simulink model "PEM_cell_validate_dynamic"  (R2025b)
settings: Solver=ode23t  StartTime=0.0  StopTime=29988  RelTol=1e-3
values from neighbouring files (symbols this model uses):
  Active_Area = 17.64    [PV_PEM_direct_battery_active.m]    (also in PV_PEM_direct_battery_passive.m; PV_PEM_indirect_battery.m; PV_PEM_reconfigurable_battery.m; Sim_vs_meas_dynamic.m)
  Input_Time = T{:,5}    [Sim_vs_meas_dynamic.m]
  Input_Voltage = T{:,16}    [Sim_vs_meas_dynamic.m]
  Ra = 0.00177    [PV_PEM_direct_battery_active.m]    (also in PV_PEM_direct_battery_passive.m; PV_PEM_indirect_battery.m; PV_PEM_reconfigurable_battery.m; Sim_vs_meas_dynamic.m)
  Rc = 0.0005    [PV_PEM_direct_battery_active.m]    (also in PV_PEM_direct_battery_passive.m; PV_PEM_indirect_battery.m; PV_PEM_reconfigurable_battery.m; Sim_vs_meas_dynamic.m)
  Rint = 0.008673    [PV_PEM_direct_battery_active.m]    (also in PV_PEM_direct_battery_passive.m; PV_PEM_indirect_battery.m; PV_PEM_reconfigurable_battery.m; Sim_vs_meas_dynamic.m)
  Vint = 1.475841    [PV_PEM_direct_battery_active.m]    (also in PV_PEM_direct_battery_passive.m; PV_PEM_indirect_battery.m; PV_PEM_reconfigurable_battery.m; Sim_vs_meas_dynamic.m)
libraries: fl_lib x15, nesl_utility x9, simulink x2
settings Model: Creator=hanna  LastModifiedBy=hanna
settings DataIOCC: SignalLogging=off  StreamToWks=off  ReturnWorkspaceOutputs=off
settings DebuggingCC: SaveWithParameterizedLinksMsg=none

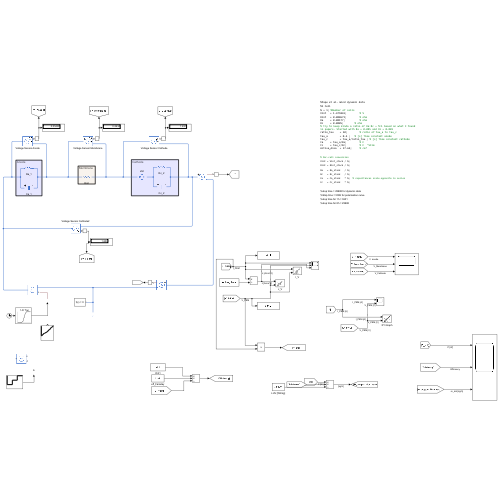
[thumbnail: Simulink's stored preview of the top-level diagram]
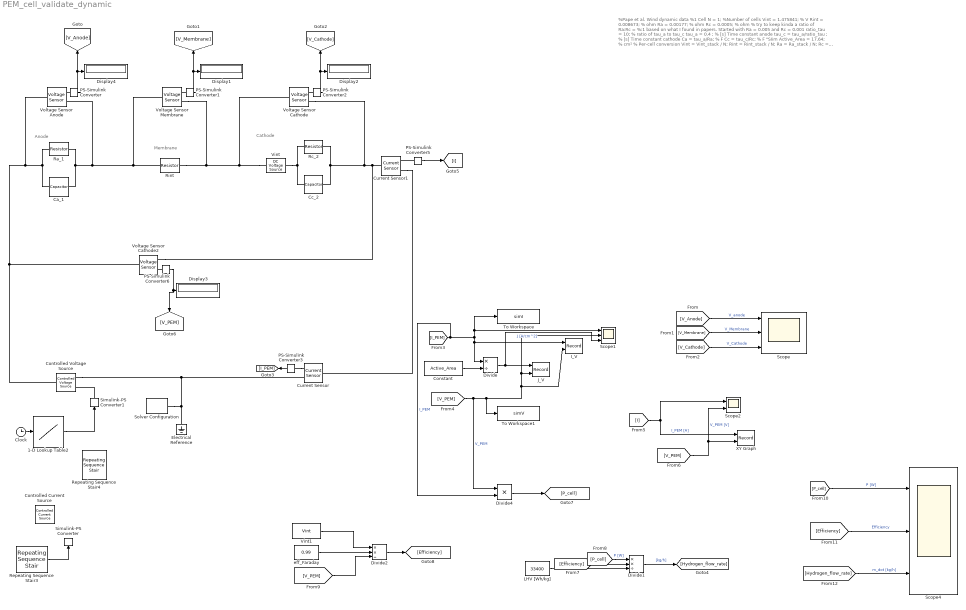
== system PEM_cell_validate_dynamic ==
  note: %Pape et al. Wind dynamic data
      | %1 Cell
      | N = 1; %Number of cells
      | Vint = 1.475841; % V
      | Rint = 0.008673; % ohm
      | Ra = 0.00177; % ohm
      | Rc = 0.0005; % ohm
      | % try to keep kinda a ratio of Ra:Rc = %:1 based on what I found in papers. Started with Ra = 0.005 and Rc = 0.001
      | ratio_tau = 10; % ratio of tau_a to tau_c
      | tau_a = 0.4 ; % [s] Time constant anode
      | tau_c = tau_a/ratio_tau ; % [s] Time constant cathode
      | Ca = tau_a/Ra; % F
      | Cc = tau_c/Rc; % F "SIim
      | Active_Area = 17.64; % cm²
      |
      | % Per-cell conversion
      | Vint = Vint_stack / N;
      | Rint = Rint_stack / N;
      | Ra = Ra_stack / N;
      | Rc = Rc_stack / N;
      | Ca = Ca_stack * N; % capacitances scale opposite in series
      | Cc = Cc_stack * N;
      |
      | %stop time = 29988 for dynamic data
      | %Stop time = 5099 for polarisation curve
      | %stop time for 1h = 3601
      | %stop time for 8h = 29988
  note: Cathode
  note: Anode
  note: Membrane
  1-D Lookup Table2 : Lookup_n-D  NumberOfTableDimensions=1  BreakpointsForDimension1=Input_Time  Table=Input_Voltage  InternalRulePriority=Speed  RndMeth=Simplest
  Ca_1 : fl_lib/Electrical/Electrical Elements/Capacitor  c=Ca F  r=1e-6 Ohm  g=0 1/Ohm  i_specify=off  i_priority=None  i=0 A  i_nominal_specify=off  i_nominal_value=1  i_nominal_unit=A  v_specify=off  v_priority=None  v=0 V  v_nominal_specify=off  v_nominal_value=1  v_nominal_unit=V  vc_specify=off  vc_priority=High  vc=0 V  vc_nominal_specify=off  vc_nominal_value=1  vc_nominal_unit=V
  Cc_2 : fl_lib/Electrical/Electrical Elements/Capacitor  c=Cc F  r=1e-6 Ohm  g=0 1/Ohm  i_specify=off  i_priority=None  i=0 A  i_nominal_specify=off  i_nominal_value=1  i_nominal_unit=A  v_specify=off  v_priority=None  v=0 V  v_nominal_specify=off  v_nominal_value=1  v_nominal_unit=V  vc_specify=off  vc_priority=High  vc=0 V  vc_nominal_specify=off  vc_nominal_value=1  vc_nominal_unit=V
  Clock : Clock
  Constant : Constant  Value=Active_Area
  Controlled Current Source : fl_lib/Electrical/Electrical Sources/Controlled Current Source
  Controlled Voltage Source : fl_lib/Electrical/Electrical Sources/Controlled Voltage Source
  Current Sensor : fl_lib/Electrical/Electrical Sensors/Current Sensor
  Current Sensor1 : fl_lib/Electrical/Electrical Sensors/Current Sensor
  Display{1..4} (4 alike) : Display
  Divide : Product  Inputs=*/
  Divide1 : Product  Inputs=**/
  Divide2 : Product  Inputs=**/
  Divide4 : Product  Inputs=**
  Electrical Reference : fl_lib/Electrical/Electrical Elements/Electrical Reference
  I_V : Record  NumPorts=2.0  FileSettingsInternal="{\"entries\":[{\"content\":{\"excelSettings\":{\"content\":{},\"type\":\"Streamout.ExcelSettings\"},\"parquetSettings\":{\"content\":{},\"type\":\"Streamout.ParquetSettings\"}},\"type\":\"Streamout.FileSettingStorage\",\"uuid\":\"\"}],\"packageUris\":[\"http:\\/\\/schema.mathworks.com\\/mf0\\/streamout_blocks\\/R2020a\"],\"version\":\"1.0\"}"  FrameSettings=[0, 0]  Layout=[1 1]  SignalsInternal="{\"entries\":[{\"content\":{\"signals\":[{\"content\":{\"blockPath\":[],\"dimensions\":[1],\"domain\":\"\",\"lineColor\":\"#ff6929\",\"lineWidth\":2,\"plots\":[ 1 ],\"port\":1,\"sid\":[\"\"],\"signalID\":1,\"signalName\":\"I_PEM\"},\"type\":\"RecordBlkView.Signal\",\"uuid\":\"\"},{\"content\":{\"blockPath\":[],\"dimensions\":[1],\"domain\":\"\",\"lineColor\":\"#64d413\",\"lineWidth\":2,\"plots\":[ 1 ],\"port\":2,\"sid\":[\"\"],\"signalID\":2,\"signalName\":\"V_PEM\"},\"type\":\"RecordBlkView.Signal\",\"uuid\":\"\"}]},\"type\":\"RecordBlkView.InputSignals\",\"uuid\":\"\"}],\"packageUris\":[\"http:\\/\\/schema.mathworks.com\\/mf0\\/streamout_blocks\\/R2020a\"],\"version\":\"1.0\"}"  VisualizationBindings="{\"xyplotplugin\":{\"info\":[{\"series\":[{\"bindingParametersList\":[{\"parameter\":\"X-Axis\",\"signalID\":1,\"signalName\":\"I_PEM\"},{\"parameter\":\"Y-Axis\",\"signalID\":2,\"signalName\":\"V_PEM\"}],\"seriesID\":0}],\"subplotID\":1}]}}"  CompatibilityTag=XY
  J_V : Record  NumPorts=2.0  FileSettingsInternal="{\"entries\":[{\"content\":{\"excelSettings\":{\"content\":{},\"type\":\"Streamout.ExcelSettings\"},\"parquetSettings\":{\"content\":{},\"type\":\"Streamout.ParquetSettings\"}},\"type\":\"Streamout.FileSettingStorage\",\"uuid\":\"\"}],\"packageUris\":[\"http:\\/\\/schema.mathworks.com\\/mf0\\/streamout_blocks\\/R2020a\"],\"version\":\"1.0\"}"  FrameSettings=[0, 0]  Layout=[1 1]  SignalsInternal="{\"entries\":[{\"content\":{\"signals\":[{\"content\":{\"blockPath\":[],\"dimensions\":[1],\"domain\":\"\",\"lineColor\":\"#a2142f\",\"plots\":[ 1 ],\"port\":1,\"sid\":[\"\"],\"signalID\":1,\"signalName\":\"J [A\\/cm^2]\"},\"type\":\"RecordBlkView.Signal\",\"uuid\":\"\"},{\"content\":{\"blockPath\":[],\"dimensions\":[1],\"domain\":\"\",\"lineColor\":\"#139fff\",\"plots\":[ 1 ],\"port\":2,\"sid\":[\"\"],\"signalID\":2,\"signalName\":\"V_PEM\"},\"type\":\"RecordBlkView.Signal\",\"uuid\":\"\"}]},\"type\":\"RecordBlkView.InputSignals\",\"uuid\":\"\"}],\"packageUris\":[\"http:\\/\\/schema.mathworks.com\\/mf0\\/streamout_blocks\\/R2020a\"],\"version\":\"1.0\"}"  VisualizationBindings="{\"xyplotplugin\":{\"info\":[{\"series\":[{\"bindingParametersList\":[{\"parameter\":\"X-Axis\",\"signalID\":1,\"signalName\":\"J [A\\/cm^2]\"},{\"parameter\":\"Y-Axis\",\"signalID\":2,\"signalName\":\"V_PEM\"}],\"seriesID\":0}],\"subplotID\":1}]}}"  CompatibilityTag=XY
  LHV [Wh/kg] : Constant  Value=33400
  PS-Simulink Converter{,1..3,5..6} (6 alike) : nesl_utility/PS-Simulink Converter  PhysicalDomain=network_engine_domain  SubClassName=ps_output  LeftPortType=input  RightPortType=output  PseudoPeriodic=off  Frequencies=[]  VectorFormat=inherit  Unit=inherit  AffineConversion=off
  Ra_1 : fl_lib/Electrical/Electrical Elements/Resistor  R=Ra Ohm  i_specify=off  i_priority=None  i=0 A  i_nominal_specify=off  i_nominal_value=1  i_nominal_unit=A  v_specify=off  v_priority=None  v=0 V  v_nominal_specify=off  v_nominal_value=1  v_nominal_unit=V
  Rc_2 : fl_lib/Electrical/Electrical Elements/Resistor  R=Rc Ohm  i_specify=off  i_priority=None  i=0 A  i_nominal_specify=off  i_nominal_value=1  i_nominal_unit=A  v_specify=off  v_priority=None  v=0 V  v_nominal_specify=off  v_nominal_value=1  v_nominal_unit=V
  Repeating Sequence Stair3 : simulink/Sources/Repeating Sequence Stair  OutValues=[10,30,50]  tsamp=50  OutMin=[]  OutMax=[]  OutDataTypeStr=double  OutputDataTypeScalingMode=double  OutDataType=fixdt(0,8)  ConRadixGroup=Best Precision: Vector-wise  OutScaling=2^-12
  Repeating Sequence Stair4 : simulink/Sources/Repeating Sequence Stair  OutValues=[1.3, 1.35, 1.4, 1.45, 1.48, 1.5 1.53, 1.55, 1.6, 1.65, 1.7, 1.75, 1.8, 1.85, 1.9, 1.95, 2.0]  tsamp=300  OutMin=[]  OutMax=[]  OutDataTypeStr=double  OutputDataTypeScalingMode=double  OutDataType=fixdt(0,8)  ConRadixGroup=Best Precision: Vector-wise  OutScaling=2^-12
  Rint : fl_lib/Electrical/Electrical Elements/Resistor  R=Rint Ohm  i_specify=off  i_priority=None  i=0 A  i_nominal_specify=off  i_nominal_value=1  i_nominal_unit=A  v_specify=off  v_priority=None  v=0 V  v_nominal_specify=off  v_nominal_value=1  v_nominal_unit=V
  Scope : Scope  NumInputPorts=3
      settings: ActiveDisplayYMinimum=-0.025574999999999994  ActiveDisplayYMaximum=0.23017500000000002  DataLoggingVariableName=ScopeData3
  Scope1 : Scope  NumInputPorts=3
      settings: ActiveDisplayYMinimum=-4.9864735642117983  ActiveDisplayYMaximum=53.61689280920104  DataLoggingVariableName=ScopeData2
  Scope2 : Scope  NumInputPorts=2
      settings: ActiveDisplayYMinimum=-5.9214977117401686  ActiveDisplayYMaximum=31.360438509949088  DataLoggingVariableName=ScopeData4
  Scope4 : Scope  NumInputPorts=3
      settings: ActiveDisplayYMinimum=-10.468413522145397  ActiveDisplayYMaximum=107.19756935479828
  Simulink-PS Converter : nesl_utility/Simulink-PS Converter  PhysicalDomain=network_engine_domain  SubClassName=ps_input  LeftPortType=input  RightPortType=output  PseudoPeriodic=off  Frequencies=[]  NoiseDistribution=none  NoiseParameters=[]  Unit=1  AffineConversion=off  FilteringAndDerivatives=provide  SimscapeFilterOrder=1  InputFilterTimeConstant=0.001  UdotUserProvided=0
  Simulink-PS Converter1 : nesl_utility/Simulink-PS Converter  PhysicalDomain=network_engine_domain  SubClassName=ps_input  LeftPortType=input  RightPortType=output  PseudoPeriodic=off  Frequencies=[]  NoiseDistribution=none  NoiseParameters=[]  Unit=1  AffineConversion=off  FilteringAndDerivatives=provide  SimscapeFilterOrder=1  InputFilterTimeConstant=0.001  UdotUserProvided=0
  Solver Configuration : nesl_utility/Solver Configuration  PhysicalDomain=network_engine_domain  SubClassName=solver  LeftPortType=input  RightPortType=generic  Tones=[]  Harmonics=[]  SimulateNoise=off  Profile=off  UseLocalSampling=off  EnableSwitchedLinearOptims=on  FrequencyDomain=off  UseCCode=off  RelTol=0.001  AbsTol=0.001  MinStep=1e-09  ToWorkspace=off  RevertToSquareIcSolve=off  NumHomotopyIterations=100  PhasorMode=off  PhasorModeNumHarmonics=1  ConsistencySolver=NEWTON_XTOL_AFTER_FTOL  IndexReductionMethod=DerivativeReplacement  DoDC=off  ResidualTolerance=1e-09  ConsistencyTolSource=GLOBAL  ConsistencyAbsTol=0.001  ConsistencyRelTol=0.001  ConsistencyTolFactor=0.001  UseLocalSolver=off  LocalSolverChoice=NE_BACKWARD_EULER_ADVANCER  ResolveIndetEquations=on  FunctionEvalNumThread=1  LocalSolverSampleTime=0.001  DoFixedCost=off  MaxNonlinIter=3  MaxModeIter=2  ComputeImpulses=off  ImpulseIterations=2  LinearAlgebra=auto  LinearAlgebraNumThread=0  EquationFormulation=NE_TIME_EF  DelaysMemoryBudget=1024  AutomaticFiltering=on  FilteringTimeConstant=0.001  PartitionStorageMethod=AS_NEEDED  PartitionMemoryBudget=1024  PartitionMethod=ROBUST  MultibodyUseLocalSolver=off  MultibodyLocalSolverChoice=ODE1  MultibodyLocalSolverSampleTime=0.001
  To Workspace : ToWorkspace  VariableName=simI  SaveFormat=Timeseries  SampleTime=0.1
  To Workspace1 : ToWorkspace  VariableName=simV  SaveFormat=Timeseries  SampleTime=0.1
  Vint : fl_lib/Electrical/Electrical Sources/DC Voltage Source  v0=Vint V
  Vint1 : Constant  Value=Vint
  Voltage Sensor Anode : fl_lib/Electrical/Electrical Sensors/Voltage Sensor
  Voltage Sensor Cathode : fl_lib/Electrical/Electrical Sensors/Voltage Sensor
  Voltage Sensor Cathode2 : fl_lib/Electrical/Electrical Sensors/Voltage Sensor
  Voltage Sensor Membrane : fl_lib/Electrical/Electrical Sensors/Voltage Sensor
  XY Graph : Record  NumPorts=2.0  FileSettingsInternal="{\"entries\":[{\"content\":{\"excelSettings\":{\"content\":{},\"type\":\"Streamout.ExcelSettings\"},\"parquetSettings\":{\"content\":{},\"type\":\"Streamout.ParquetSettings\"}},\"type\":\"Streamout.FileSettingStorage\",\"uuid\":\"\"}],\"packageUris\":[\"http:\\/\\/schema.mathworks.com\\/mf0\\/streamout_blocks\\/R2020a\"],\"version\":\"1.0\"}"  FrameSettings=[0, 0]  Layout=[1 1]  SignalsInternal="{\"entries\":[{\"content\":{\"signals\":[{\"content\":{\"blockPath\":[],\"dimensions\":[1],\"domain\":\"\",\"lineColor\":\"#a2142f\",\"lineWidth\":2,\"plots\":[ 1 ],\"port\":1,\"sid\":[\"\"],\"signalID\":1,\"signalName\":\"I_PEM [A]\"},\"type\":\"RecordBlkView.Signal\",\"uuid\":\"\"},{\"content\":{\"blockPath\":[],\"dimensions\":[1],\"domain\":\"\",\"lineColor\":\"#139fff\",\"lineWidth\":2,\"plots\":[ 1 ],\"port\":2,\"sid\":[\"\"],\"signalID\":2,\"signalName\":\"V_PEM [V]\"},\"type\":\"RecordBlkView.Signal\",\"uuid\":\"\"}]},\"type\":\"RecordBlkView.InputSignals\",\"uuid\":\"\"}],\"packageUris\":[\"http:\\/\\/schema.mathworks.com\\/mf0\\/streamout_blocks\\/R2020a\"],\"version\":\"1.0\"}"  VisualizationBindings="{\"xyplotplugin\":{\"info\":[{\"series\":[{\"bindingParametersList\":[{\"parameter\":\"X-Axis\",\"signalID\":1,\"signalName\":\"I_PEM [A]\"},{\"parameter\":\"Y-Axis\",\"signalID\":2,\"signalName\":\"V_PEM [V]\"}],\"seriesID\":0}],\"subplotID\":1}]}}"  CompatibilityTag=XY
  eff_Faraday : Constant  Value=0.99
  wires:
  [V_PEM] -> Divide4/1, To Workspace1/1, Scope1/2, J_V/2, I_V/2  "V_PEM"
  PS-Simulink Converter3/1 -> [I_PEM]
  [I_PEM] -> Scope1/1, To Workspace/1, Divide/1, I_V/1, Divide4/2  "I_PEM"
  Divide/1 -> Scope1/3, J_V/1  "J [A/cm^2]"
  Constant/1 -> Divide/2
  [V_Anode] -> Scope/1  "V_anode"
  PS-Simulink Converter6/1 -> [V_PEM], Display3/1
  [V_Membrane] -> Scope/2  "V_Membrane"
  PS-Simulink Converter5/1 -> [I]
  PS-Simulink Converter/1 -> [V_Anode], Display4/1
  PS-Simulink Converter1/1 -> [V_Membrane], Display1/1
  [V_PEM] -> Scope2/2, XY Graph/2  "V_PEM [V]"
  [V_Cathode] -> Scope/3  "V_Cathode"
  [I] -> Scope2/1, XY Graph/1  "I_PEM [A]"
  PS-Simulink Converter2/1 -> [V_Cathode], Display2/1
  Divide4/1 -> [P_cell]
  [P_cell] -> Divide1/1  "P [W]"
  LHV [Wh/kg]/1 -> Divide1/3
  Divide1/1 -> [Hydrogen_flow_rate]  "[kg/h]"
  [Efficiency] -> Divide1/2
  [V_PEM] -> Divide2/3
  Vint1/1 -> Divide2/1
  eff_Faraday/1 -> Divide2/2
  Divide2/1 -> [Efficiency]
  [Hydrogen_flow_rate] -> Scope4/3  "m_dot [kg/h]"
  [Efficiency] -> Scope4/2  "Efficiency"
  [P_cell] -> Scope4/1  "P [W]"
  Clock/1 -> 1-D Lookup Table2/1
  Repeating Sequence Stair3/1 -> Simulink-PS Converter/1
  1-D Lookup Table2/1 -> Simulink-PS Converter1/1
  connections:
  Electrical Reference/LConn1 -- Controlled Voltage Source/RConn2 -- Current Sensor/RConn2 -- Solver Configuration/RConn1
  PS-Simulink Converter3/LConn1 -- Current Sensor/RConn1
  Ca_1/RConn1 -- Ra_1/RConn1 -- Voltage Sensor Anode/RConn2 -- Voltage Sensor Membrane/LConn1 -- Rint/LConn1
  Current Sensor1/LConn1 -- Rc_2/RConn1 -- Cc_2/RConn1 -- Voltage Sensor Cathode/RConn2 -- Voltage Sensor Cathode2/RConn2
  Vint/LConn1 -- Rint/RConn1 -- Voltage Sensor Membrane/RConn2 -- Voltage Sensor Cathode/LConn1
  Cc_2/LConn1 -- Rc_2/LConn1 -- Vint/RConn1
  Voltage Sensor Cathode2/LConn1 -- Controlled Voltage Source/LConn1 -- Voltage Sensor Anode/LConn1 -- Ra_1/LConn1 -- Ca_1/LConn1
  Voltage Sensor Cathode2/RConn1 -- PS-Simulink Converter6/LConn1
  Voltage Sensor Cathode/RConn1 -- PS-Simulink Converter2/LConn1
  PS-Simulink Converter5/LConn1 -- Current Sensor1/RConn1
  Current Sensor1/RConn2 -- Current Sensor/LConn1
  Voltage Sensor Membrane/RConn1 -- PS-Simulink Converter1/LConn1
  Voltage Sensor Anode/RConn1 -- PS-Simulink Converter/LConn1
  Simulink-PS Converter1/RConn1 -- Controlled Voltage Source/RConn1
